simulink model "TIM"  (R2017b)
settings: Solver=VariableStepAuto  StartTime=0.0  StopTime=50  FixedStep=0.1  RelTol=1e-3
undefined symbols (not defined in the file): sigbuilder_block
(part 2 of 2)

== stateflow chart TIM/Baler/BalerMode1 ==
  state SensorsLogic [parallel]
    settings: executionOrder=1
    state BothSrsWork
      entry: BalerMode=3;
      SysReconfigReq=0;
    state FirstSrFail
      entry:  BalerMode=3.2;
      SysReconfigReq=0;
    state BotheFail
      entry:  BalerMode=1;
      SysReconfigReq=1;
    state SecondSrFail [commented out]
      entry:  BalerMode=2;
      SysReconfigReq=1.2;
    BothSrsWork -> FirstSrFail : [RObstSr_isBroken(RSr1) ]
    (default) -> BothSrsWork
    FirstSrFail -> BothSrsWork [order 2] : [~(RObstSr_isBroken(RSr1))]
    BothSrsWork -> SecondSrFail [commented out] : [RObstSr_isBroken(RSr2)]
    SecondSrFail -> BothSrsWork [commented out] : [~RObstSr_isBroken(RSr2)]
    BotheFail -> BothSrsWork [order 1] : [~(RObstSr_isBroken(RSr1))&&~(RObstSr_isBroken(RSr2))]
    BotheFail -> FirstSrFail [order 2] : [~(RObstSr_isBroken(RSr2))]
    FirstSrFail -> BotheFail [order 1] : [(RObstSr_isBroken(RSr2))]
    SecondSrFail -> BotheFail [commented out] : [RObstSr_isBroken(RSr1)]
    BotheFail -> SecondSrFail [commented out] : [~RObstSr_isBroken(RSr1)]
  state BalerLogic [parallel]
    settings: executionOrder=2
    state Auto
      entry: SysModeOut=3 ;
      ِ
      state Auto3
        entry:BalerCfgMode=3.2;
        AutoCfg_2=true;
        exit:AutoCfg_2=false;
      state Auto1
        entry:BalerCfgMode=3.1;
        AutoCfg_1=true;
        exit:AutoCfg_1=false;
        ِ
      Auto1 -> Auto3 : [ BalerMode==3.2]
      (default) -> Auto1
    state SemiAuto
      entry: SysModeOut=2;
      BalerCfgMode=2;
      SemiAutoCfg=true;
      exit:SemiAutoCfg=false;
    state Manual
      entry: SysModeOut=1;
      BalerCfgMode=1;
      ManualCfg=true;
      exit: ManualCfg=false;
    Manual -> Auto [order 2] : [ModeInput==3]
    Manual -> SemiAuto [order 1] : [ModeInput==2&&(BalerMode~=1)]
    (default) -> Manual
    SemiAuto -> Auto [order 1] : [ModeInput==3]
    SemiAuto -> Manual [order 2] : [ModeInput==1]
    Auto -> SemiAuto [order 3] : [ModeInput==2]
    Auto -> Manual [order 1] : [ModeInput==1]
    Auto -> SemiAuto [order 2] : [( ModeInput==2)]
  data: obst function_input; status function_output; ModeInput input; SysModeOut output; RSr1 input; RSr2 input; BalerCfgMode output; SysReconfigReq output; AutoCfg_1 output; AutoCfg_2 output; SemiAutoCfg output; BalerMode local; ManualCfg output boolean
  function status=RObstSr_isBroken(obst):
    | function status=RObstSr_isBroken(obst)
    |  
    | if ((obst==1)||(obst==0))
    | 
    | status=false;
    | else
    |     status=true;
    | end

== stateflow chart TIM/Tractor/TractorMode ==
  state Manual
    entry: SysModeOut=1;
    ManualCfg=true;
    exit:ManualCfg=false;
    UrgentSpeed=0;
  state SemiAuto
    entry: SysModeOut=2;
    SemiAutoCfg=true;
    exit:SemiAutoCfg=false;
  state Auto
    entry: SysModeOut=3;
    AutoCfg=true;
    exit:AutoCfg=false;
  Manual -> Auto [order 2] : [(ModeInput==3)&&(SysReconfigReq~=1)]
  Auto -> SemiAuto [order 2] : [(ModeInput==2) || (FrontObsSr_isBroken(Fobst))]{ AutoCfg=false}
  (default) -> Manual
  Manual -> SemiAuto [order 1] : [ModeInput==2&&((SysReconfigReq~=1)&&(SysReconfigReq~=1.2))]
  SemiAuto -> Manual [order 2] : [(ModeInput==1)||(SysReconfigReq==1)]{UrgentSpeed=1;}
  SemiAuto -> Auto [order 1] : [(ModeInput==3)&&(~FrontObsSr_isBroken(Fobst))]
  Auto -> Manual [order 1] : [(ModeInput==1)||(SysReconfigReq==1)]{UrgentSpeed=1;}
  data: FobstValue function_input; status function_output; ModeInput input; SysModeOut output; Fobst input; AutoCfg output boolean; SemiAutoCfg output boolean; ManualCfg output boolean; SysReconfigReq input; UrgentSpeed output
  function status = FrontObsSr_isBroken(FobstValue):
    | function status=FrontObsSr_isBroken(FobstValue)
    | 
    | if ((FobstValue==1)||(FobstValue==0))
    | 
    | status=false;
    | else
    |     status=true;
    | end

== stateflow chart TIM/Tractor/Auto_Cfg SubSystem/SpeedController/Chart ==
  state S0
    entry:Speed=0;
    du:Speed = Speed +1;
  state S4
    du:Speed= Speed +1;
  state S1
    du:Speed = TSpeed;
  state S3
    du:Speed =0;
  state S2
    du:Speed = Speed - 1;
  state S5
    du:Speed= 8;
  (default) -> S0
  S3 -> S4 : [FObstSr==0&&(BaleSize==0)]
  S4 -> S1 [order 1] : [Speed==8]
  S0 -> S1 : [Speed==8]
  S4 -> S2 [order 2] : [FObstSr==1]
  S2 -> S4 [order 1] : [FObstSr==0]
  S5 -> S4 [order 2] : [FObstSr==0]
  S1 -> S2 : [FObstSr==1||(BaleSize==1)]
  (junction 26) -> S3 [order 1] : [ObstDist<=2.5||(BaleSize==2)]
  S5 -> S3 [order 1] : [ObstDist<=2.5||(BaleSize==2)]
  S2 -> (junction 26) [order 2]
  (junction 26) -> S5 [order 2] : [Speed<9&&(~(ObstDist<=2.5))]
  data: CSpeed input double; TSpeed input; BaleSize input; FObstSr input; Speed output; ObstDist input

== stateflow chart TIM/SwathScanner/Chart ==
  state AutoCfg
    state Auto1
      entry: SysModeOut=3.1;
      AutoCfg1=true;
      exit: AutoCfg1=false;
    state Auto2
      entry: SysModeOut=3.2;
      AutoCfg2=true;
      exit:AutoCfg2=false;
    (default) -> (junction 63) [commented out]
    (junction 63) -> Auto2 [commented out] : [isBroken(SpSr1)==true]
    (junction 63) -> Auto1 [commented out] : [[isBroken(SpSr1)==false]]
    Auto1 -> Auto2 : [isBroken(SpSr1)==true]
    (default) -> Auto1
  state SemiAuto
    entry: SysModeOut=2;
    SemiAutoCfg=true;
    exit:SemiAutoCfg=false;
  state Manual
    entry: SysModeOut=1;
    ManualCfg=true;
    exit:ManualCfg=false;
  Manual -> AutoCfg [order 2] : [ModeInput==3]
  AutoCfg -> SemiAuto [order 1] : [ModeInput==2]
  Manual -> SemiAuto [order 1] : [ModeInput==2]
  (default) -> Manual
  SemiAuto -> AutoCfg [order 1] : [ModeInput==3]
  SemiAuto -> Manual [order 2] : [ModeInput==1]
  AutoCfg -> Manual [order 2] : [ModeInput==1]
  data: Speed function_input; status function_output; ModeInput input; SysModeOut output; AutoCfg1 output boolean; AutoCfg2 output boolean; SemiAutoCfg output boolean; SpSr1 input; ManualCfg output boolean
  function status=isBroken(Speed):
    | function status=isBroken(Speed)
    | 
    | if ((Speed>20)||(Speed<0))
    | 
    | status=true;
    | else
    |     status=false;
    | end

== matlab function TIM/SwathScanner/Auto_1_Cfg Subsystem/CalcVolFlowRate 1/MATLAB Function ==
  data: speed input; y output; area input
function y = fcn(speed, area)

y = speed*area;

== matlab function TIM/SwathScanner/Auto_2_Cfg Subsystem/CalcVolFlowRate 1/MATLAB Function ==
  data: speed input; y output; area input
function y = fcn(speed, area)

y = speed*area;

== matlab function TIM/Tractor/SemiAuto_Cfg SubSystem/SpeedController/setSpeed ==
  data: Cspeed input; y output; Tspeed input; BaleSize input; FrontObstSr input
function y = fcn(Cspeed, Tspeed,BaleSize, FrontObstSr)

if(BaleSize==2 || FrontObstSr==1)
    y = (Cspeed-(Cspeed-Tspeed))*0;


elseif(BaleSize==1)
y = ((Cspeed-(Cspeed-Tspeed))*0.50);
else
   y = (Cspeed-(Cspeed-Tspeed)); 
end

== matlab function TIM/Tractor/ManualCfg SubSystem/SpeedController/setSpeed ==
  data: Cspeed input; y output; SpBedalAngl input; StopReq input; Urgent input; UserPresent input
function y = fcn(Cspeed, SpBedalAngl, StopReq,Urgent, UserPresent)

if(StopReq==1)
    y = 0;
elseif((Urgent==1)&&(UserPresent==0))
    y = 0;
else
   y = (Cspeed-(Cspeed-(4*SpBedalAngl))); 
end

== matlab function TIM/Baler/AutoCfg_2 Subsystem/CalcTargetAngel ==
  data: SWL input; TargetAngle output
function TargetAngle = fcn(SWL)

  
TargetAngle = 3*SWL;
end

== matlab function TIM/Baler/AutoCfg_2 Subsystem/CalcTargetSpeed/MATLAB Function ==
  data: u input; TargetSpeed output
function TargetSpeed = fcn(u)

  
TargetSpeed = -.10*u+20;
end

== matlab function TIM/Baler/AutoCfg_2 Subsystem/RearDoorControl/CloseRearDoor ==
  data: DoorStatus input; y output; BaleOutSr input
function y = fcn(DoorStatus, BaleOutSr)
if (DoorStatus==1 &&BaleOutSr==1)
y = 0;
else
 y=DoorStatus;
    
end

== matlab function TIM/Baler/AutoCfg_2 Subsystem/RearDoorControl/OpenRearDoorFunction ==
  data: StopSignal input; Y output; BaleSize input; RearObstSr input

function Y = fcn(StopSignal,BaleSize,RearObstSr)

if (StopSignal==1 && BaleSize==2 && RearObstSr==0)
    Y =1;
else
    
    Y=0;
    
end

== matlab function TIM/SwathScanner/SemiAuto_Cfg Subsystem/CalcVolFlowRate 1/MATLAB Function ==
  data: speed input; y output; area input
function y = fcn(speed, area)

y = speed*area;

== matlab function TIM/Baler/SemiAutoCfg Subsystem/CalcTargetSpeed/MATLAB Function ==
  data: u input; TargetSpeed output
function TargetSpeed = fcn(u)

  
TargetSpeed = -.10*u+20;
end

== matlab function TIM/Baler/SemiAutoCfg Subsystem/RearDoorControl/CloseRearDoor ==
  data: DoorStatus input; y output; BaleOutSr input
function y = fcn(DoorStatus, BaleOutSr)
if (DoorStatus==1 &&BaleOutSr==1)
y = 0;
else
 y=DoorStatus;
    
end

== matlab function TIM/Baler/SemiAutoCfg Subsystem/RearDoorControl/OpenRearDoorFunction ==
  data: StopSignal input; Y output; BaleSize input; RearObstSr input

function Y = fcn(StopSignal,BaleSize,RearObstSr)

if (StopSignal==1 && BaleSize==2 && RearObstSr==0)
    Y =1;
else
    
    Y=0;
    
end

== matlab function TIM/Tractor/ManualCfg SubSystem/setStAngle ==
  data: TAngle input; CAngle output
function CAngle = fcn( TAngle )


   CAngle = 3*TAngle; 
end

== matlab function TIM/Tractor/Auto_Cfg SubSystem/setStAngle ==
  data: TAngle input; CAngle output
function CAngle = fcn( TAngle )


   CAngle = TAngle; 
end

== matlab function TIM/Tractor/SemiAuto_Cfg SubSystem/setStAngle ==
  data: TAngle input; CAngle output
function CAngle = fcn( TAngle )


   CAngle = 3*TAngle; 
end
